simulink model "LegoLab (5)"  (R2023a)
settings: Solver=FixedStepAuto  StartTime=0.0  StopTime=10.0  RelTol=1e-3  EnableMultiTasking=on
libraries: legoev3lib x14, simulink x1
settings Model: ExtModeTrigDuration=2  Creator=odins  LastModifiedBy=augus
settings SolverCC: PositivePriorityOrder=on  AutoInsertRateTranBlk=on
settings OptimizationCC: EnhancedBackFolding=on  PassReuseOutputArgsAs=Individual arguments  ZeroExternalMemoryAtStartup=off  ZeroInternalMemoryAtStartup=off  MaxStackSize=64  OptimizeBlockOrder=speed  DifferentSizesBufferReuse=on  OptimizationCustomize=off  EfficientTunableParamExpr=on
settings DebuggingCC: ParameterTunabilityLossMsg=error
settings HardwareCC: ProdBitPerPointer=32  ProdBitPerSizeT=32  ProdBitPerPtrDiffT=32  ProdLargestAtomicInteger=Long  ProdWordSize=32  ProdHWDeviceType=ARM Compatible->ARM 9  UseEmbeddedCoderFeatures=off  UseSimulinkCoderFeatures=off
settings SFSimCC: MATLABDynamicMemAlloc=off
settings RTWCC: Description=Embedded Coder  SystemTargetFile=ert.tlc  HardwareBoard=LEGO MINDSTORMS EV3  TLCOptions="-aInlineSetEventsForThisBaseRateFcn=TLC_FALSE -aSuppressMultiTaskScheduler=TLC_FALSE  -aRateBasedStepFcn=0"  TemplateMakefile=ert_default_tmf  Toolchain=Sourcery G++ Lite v2009q3
settings CodeAppCC: ForceParamTrailComments=on  IgnoreCustomStorageClasses=off  OperatorAnnotations=on  SimulinkDataObjDesc=on  SFDataObjDesc=on  InsertBlockDesc=on
settings ERTTargetCC: SupportContinuousTime=on  SupportNonInlinedSFcns=on  SupportVariableSizeSignals=on  ExtModeTransport=2  ExtModeStaticAlloc=on  ExtModeMexFile=ext_xcp  ExtModeIntrfLevel=Level2 - Open

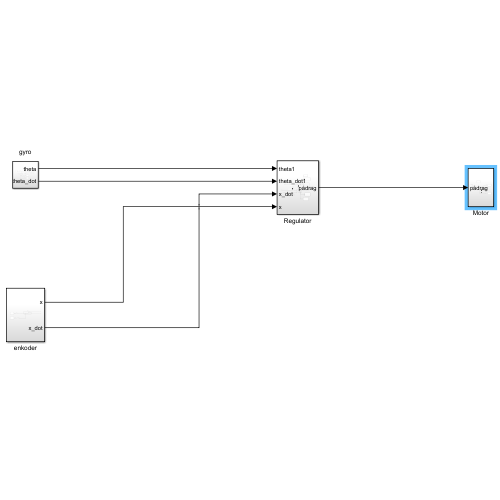
[thumbnail: Simulink's stored preview of the top-level diagram]
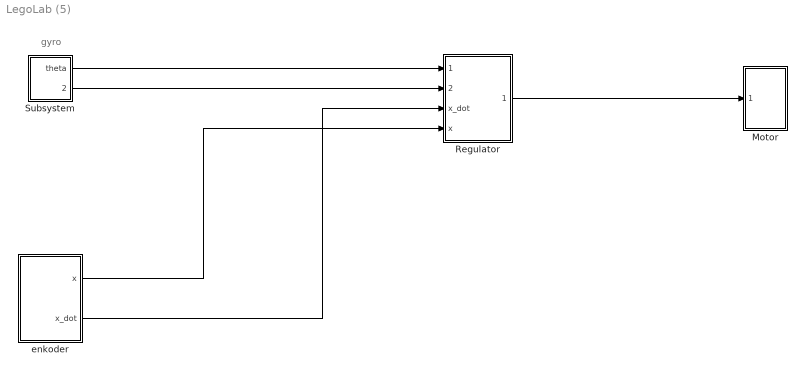
== system LegoLab (5) ==
  note: gyro
  Motor : Subsystem
  Regulator : Subsystem
  Subsystem : Subsystem
  enkoder : Subsystem
  wires:
  enkoder/1(x) -> Regulator/4(x)
  enkoder/2(x_dot) -> Regulator/3(x_dot)
  Subsystem/2(theta_dot) -> Regulator/2(theta_dot1)
  Subsystem/1(theta) -> Regulator/1(theta1)
  Regulator/1(pådrag) -> Motor/1(pådrag)

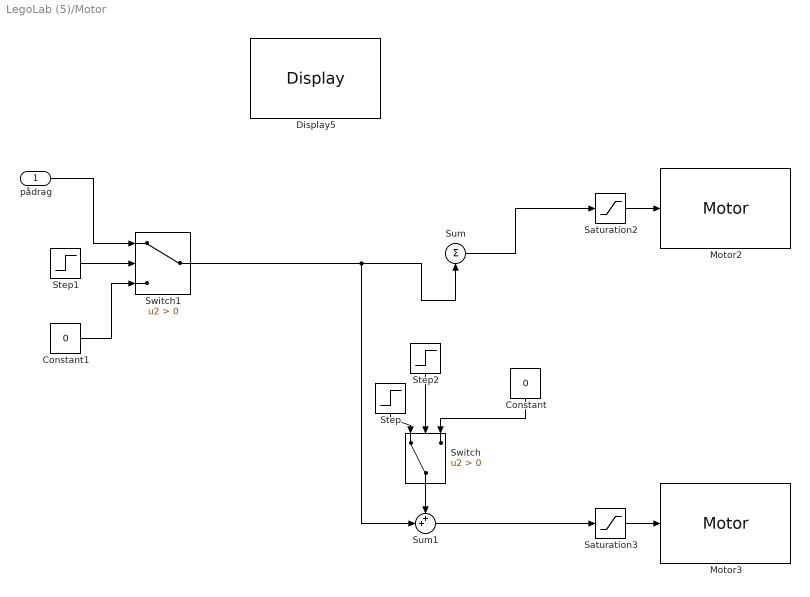
== system LegoLab (5)/Motor ==
  pådrag : Inport
  Constant : Constant  Value=0
  Constant1 : Constant  Value=0
  Display5 : legoev3lib/Display  slcdStr=padrag  slcdLine=10  slcdFormat=Decimal
  Motor2 : legoev3lib/Motor  sportNumber=A  sstopAction=Brake
  Motor3 : legoev3lib/Motor  sportNumber=D  sstopAction=Brake
  Saturation2 : Saturate  UpperLimit=100  LowerLimit=-100
  Saturation3 : Saturate  UpperLimit=100  LowerLimit=-100
  Step : Step  Time=13  Before=20  After=0  SampleTime=0
  Step1 : Step  Time=5  SampleTime=0
  Step2 : Step  Time=10  SampleTime=0
  Sum : Sum  Inputs=|+
  Sum1 : Sum  Inputs=++|
  Switch : Switch  Criteria=u2 > Threshold  SaturateOnIntegerOverflow=off  InputSameDT=off
  Switch1 : Switch  Criteria=u2 > Threshold  SaturateOnIntegerOverflow=off  InputSameDT=off
  wires:
  Switch1/1 -> Sum/1, Sum1/2
  pådrag/1 -> Switch1/1
  Saturation3/1 -> Motor3/1
  Constant1/1 -> Switch1/3
  Saturation2/1 -> Motor2/1
  Step1/1 -> Switch1/2
  Sum/1 -> Saturation2/1
  Sum1/1 -> Saturation3/1
  Step/1 -> Switch/1
  Switch/1 -> Sum1/1
  Constant/1 -> Switch/3
  Step2/1 -> Switch/2

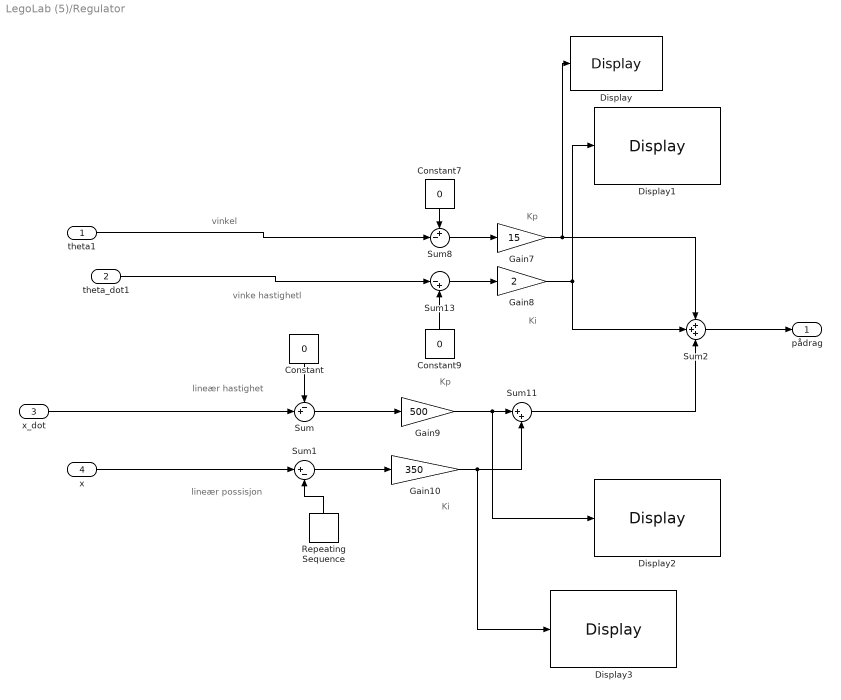
== system LegoLab (5)/Regulator ==
  note: lineær possisjon
  note: lineær hastighet
  note: vinkel
  note: vinke hastighetl
  note: Kp
  note: Ki
  note: Kp
  note: Ki
  theta1 : Inport
  theta_dot1 : Inport  Port=2
  x_dot : Inport  Port=3
  x : Inport  Port=4
  Constant : Constant  Value=0
  Constant7 : Constant  Value=0
  Constant9 : Constant  Value=0
  Display : legoev3lib/Display  slcdStr=gyro kp  slcdLine=1  slcdFormat=Decimal
  Display1 : legoev3lib/Display  slcdStr=gyro ki  slcdLine=2  slcdFormat=Decimal
  Display2 : legoev3lib/Display  slcdStr=enc kp  slcdLine=3  slcdFormat=Decimal
  Display3 : legoev3lib/Display  slcdStr=enc ki  slcdLine=4  slcdFormat=Decimal
  Gain10 : Gain  Gain=350
  Gain7 : Gain  Gain=15
  Gain8 : Gain  Gain=2
  Gain9 : Gain  Gain=500
  Repeating Sequence : simulink/Sources/Repeating Sequence  rep_seq_t=[0 5 7 10 12]  rep_seq_y=[0 0 0.25 0.25 0.25]
  Sum : Sum  Inputs=-+|
  Sum1 : Sum  Inputs=|+-
  Sum11 : Sum  Inputs=|++
  Sum13 : Sum  Inputs=|-+
  Sum2 : Sum  Inputs=+++
  Sum8 : Sum  Inputs=+-|
  pådrag : Outport
  wires:
  Gain10/1 -> Display3/1, Sum11/2
  Gain7/1 -> Sum2/1, Display/1
  Sum13/1 -> Gain8/1
  Gain9/1 -> Display2/1, Sum11/1
  Constant7/1 -> Sum8/1
  Sum11/1 -> Sum2/3
  x/1 -> Sum1/1
  Constant9/1 -> Sum13/2
  Sum8/1 -> Gain7/1
  Gain8/1 -> Sum2/2, Display1/1
  theta_dot1/1 -> Sum13/1
  theta1/1 -> Sum8/2
  Sum/1 -> Gain9/1
  Sum1/1 -> Gain10/1
  Constant/1 -> Sum/1
  Repeating Sequence/1 -> Sum1/2
  Sum2/1 -> pådrag/1
  x_dot/1 -> Sum/2

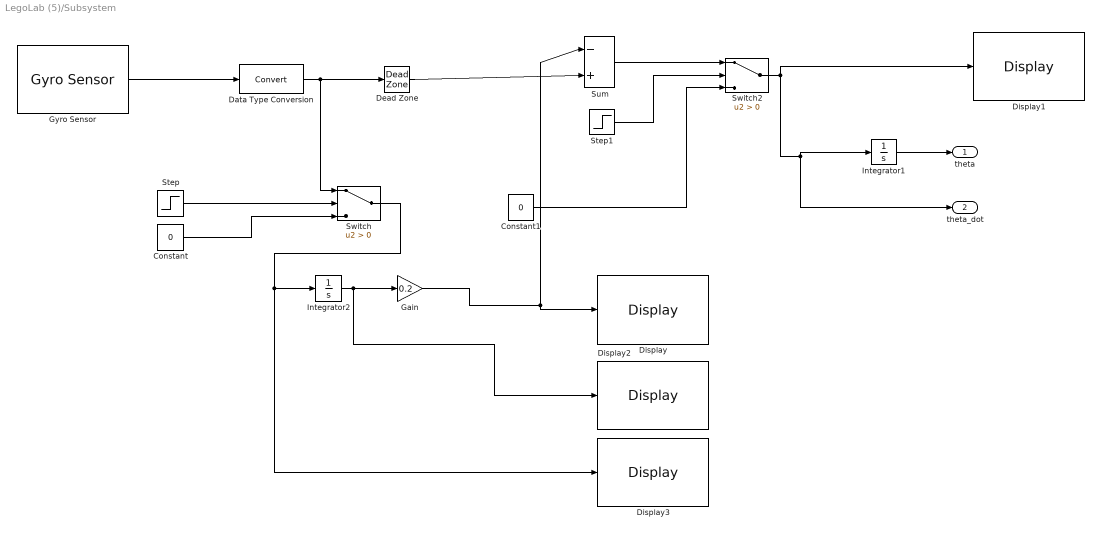
== system LegoLab (5)/Subsystem ==
  Constant : Constant  Value=0
  Constant1 : Constant  Value=0
  Data Type Conversion : DataTypeConversion  SaturateOnIntegerOverflow=off  RndMeth=Floor
  Dead Zone : DeadZone  LowerValue=-1  UpperValue=1
  Display : legoev3lib/Display  slcdStr=kalib  slcdLine=2  slcdFormat=Decimal
  Display1 : legoev3lib/Display  slcdStr=9  slcdLine=10  slcdFormat=Decimal
  Display2 : legoev3lib/Display  slcdStr=e2  slcdLine=9  slcdFormat=Decimal
  Display3 : legoev3lib/Display  slcdStr=fI  slcdLine=8  slcdFormat=Decimal
  Gain : Gain  Gain=0.2
  Gyro Sensor : legoev3lib/Gyro Sensor  portNumber=2  sampleTime=0.01
  Integrator1 : Integrator
  Integrator2 : Integrator
  Step : Step  Time=5  Before=1  After=0  SampleTime=0
  Step1 : Step  Time=5  SampleTime=0
  Sum : Sum  Inputs=|-+
  Switch : Switch  Criteria=u2 > Threshold  SaturateOnIntegerOverflow=off  InputSameDT=off
  Switch2 : Switch  Criteria=u2 > Threshold  SaturateOnIntegerOverflow=off  InputSameDT=off
  theta : Outport
  theta_dot : Outport  Port=2
  wires:
  Switch2/1 -> theta_dot/1, Integrator1/1, Display1/1
  Step1/1 -> Switch2/2
  Constant1/1 -> Switch2/3
  Step/1 -> Switch/2
  Gyro Sensor/1 -> Data Type Conversion/1
  Integrator2/1 -> Display2/1, Gain/1
  Constant/1 -> Switch/3
  Sum/1 -> Switch2/1
  Gain/1 -> Sum/1, Display/1
  Switch/1 -> Display3/1, Integrator2/1
  Integrator1/1 -> theta/1
  Data Type Conversion/1 -> Dead Zone/1, Switch/1
  Dead Zone/1 -> Sum/2

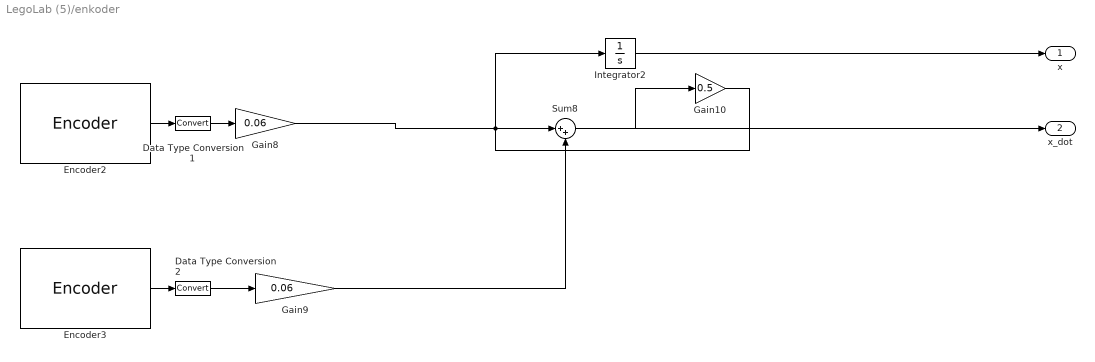
== system LegoLab (5)/enkoder ==
  Data Type Conversion1 : DataTypeConversion  SaturateOnIntegerOverflow=off  RndMeth=Floor
  Data Type Conversion2 : DataTypeConversion  SaturateOnIntegerOverflow=off  RndMeth=Floor
  Encoder2 : legoev3lib/Encoder  portNumber=A  opMode=Reset at each sample time  sampleTime=0.01
  Encoder3 : legoev3lib/Encoder  portNumber=D  opMode=Reset at each sample time  sampleTime=0.01
  Gain10 : Gain  Gain=0.5
  Gain8 : Gain  Gain=0.06
  Gain9 : Gain  Gain=0.06
  Integrator2 : Integrator
  Sum8 : Sum  Inputs=|++
  x : Outport
  x_dot : Outport  Port=2
  wires:
  Sum8/1 -> Gain10/1
  Gain9/1 -> Sum8/2
  Integrator2/1 -> x/1
  Encoder3/1 -> Data Type Conversion2/1
  Gain8/1 -> Sum8/1
  Gain10/1 -> Integrator2/1, x_dot/1
  Data Type Conversion1/1 -> Gain8/1
  Encoder2/1 -> Data Type Conversion1/1
  Data Type Conversion2/1 -> Gain9/1
